simulink model "ECE556Lab1Task7b"  (R2013b)
settings: Solver=ode45  StartTime=0.0  StopTime=.5  MaxStep=.001  RelTol=1e-3
settings Model: Creator=Ben  LastModifiedBy=Ben

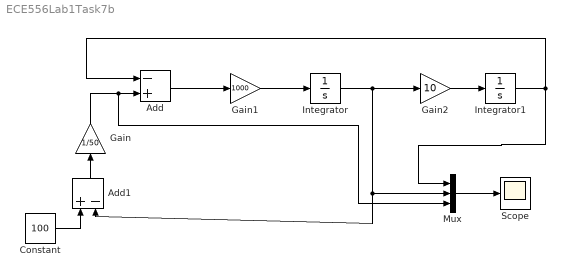
== system ECE556Lab1Task7b ==
  Add : Sum  Inputs=-+
  Add1 : Sum  Inputs=+-
  Constant : Constant  Value=100
  Gain : Gain  Gain=1/50
  Gain1 : Gain  Gain=1000
  Gain2 : Gain  Gain=10
  Integrator : Integrator
  Integrator1 : Integrator
  Mux : Mux  Inputs=3
  Scope : Scope
  wires:
  Constant/1 -> Add1/1
  Gain/1 -> Mux/3, Add/2
  Add1/1 -> Gain/1
  Add/1 -> Gain1/1
  Gain1/1 -> Integrator/1
  Integrator/1 -> Mux/2, Add1/2, Gain2/1
  Gain2/1 -> Integrator1/1
  Integrator1/1 -> Mux/1, Add/1
  Mux/1 -> Scope/1
